simulink model "Test_Counter_4bit_Cfg"  (R2023a)
settings: Solver=VariableStepAuto  StartTime=0.0  StopTime=1000.0  MaxStep=1  MinStep=1  RelTol=1e-3  EnableMultiTasking=on
libraries: simulink x2, simulink_extras x1, Counters_Lib x1
settings Model: PauseTimes=0  Creator=Jozko Mrkvicka  LastModifiedBy=Jozko Mrkvicka
settings SolverCC: InitialStep=1  AlgebraicLoopSolver=TrustRegion
settings DataIOCC: ReturnWorkspaceOutputs=off
settings OptimizationCC: LifeSpan=inf
settings DebuggingCC: UnconnectedInputMsg=warning  UnconnectedOutputMsg=warning  UnconnectedLineMsg=warning  SFUnexpectedBacktrackingDiag=warning  SFNoUnconditionalDefaultTransitionDiag=warning  ArithmeticOperatorsInVariantConditions=warning
settings ModelReferenceCC: EnableRefExpFcnMdlSchedulingChecks=on
settings SFSimCC: SimUseLocalCustomCode=off  CustomCodeUndefinedFunction=UseInterfaceOnly
settings RTWCC: RTWUseLocalCustomCode=off
settings CodeAppCC: StateflowObjectComments=on
settings GRTTargetCC: TargetLangStandard=C89/C90 (ANSI)
settings ConfigComp: CovMetricSettings=dw  CovSaveCumulativeToWorkspaceVar=on  CovSaveSingleToWorkspaceVar=on  CovExternalEMLEnable=off

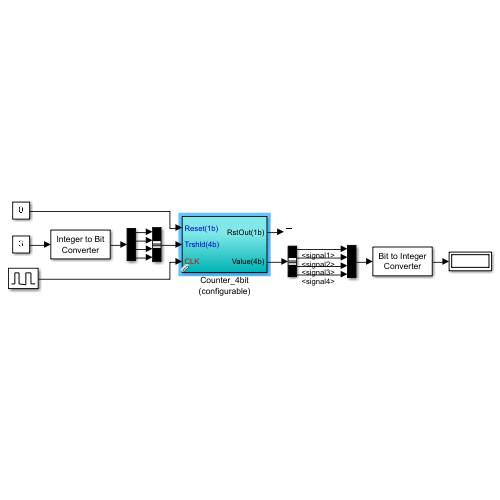
[thumbnail: Simulink's stored preview of the top-level diagram]
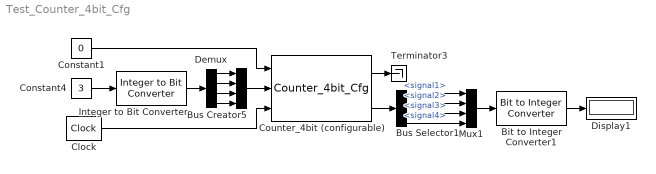
== system Test_Counter_4bit_Cfg ==
  Bit to Integer Converter1 : simulink/Logic and Bit Operations/Bit to Integer Converter  nbits=4  bitOrder=MSB first  signedOutputValues=Unsigned  outDtype=uint8  outDtypeSigned=Inherit via internal rule
      settings: LibrarySourceBlock=|
      | commutil2/Bit to Integer
      | Converter
  Bus Creator5 : BusCreator  Inputs=4
  Bus Selector1 : BusSelector  OutputSignals=signal1,signal2,signal3,signal4
  Clock : simulink_extras/Flip Flops/Clock  period=2
  Constant1 : Constant  Value=0  OutDataTypeStr=boolean
  Constant4 : Constant  Value=3
  Counter_4bit (configurable) : Counters_Lib/Counter_4bit_Cfg  SystemSampleTime=-1  VariantActivationTime=update diagram  Latency=0  AutoFrameSizeCalculation=off
  Demux : Demux
  Display1 : Display
  Integer to Bit Converter : simulink/Logic and Bit Operations/Integer to Bit Converter  nbits=4  signedInputValues=Unsigned  bitOrder=MSB first  outDtype=Inherit via internal rule
      settings: LibrarySourceBlock=|
      | commutil2/Integer to Bit
      | Converter
  Mux1 : Mux
  Terminator3 : Terminator
  wires:
  Mux1/1 -> Bit to Integer Converter1/1
  Bit to Integer Converter1/1 -> Display1/1
  Constant4/1 -> Integer to Bit Converter/1
  Integer to Bit Converter/1 -> Demux/1
  Clock/1 -> Counter_4bit (configurable)/3
  Bus Creator5/1 -> Counter_4bit (configurable)/2
  Constant1/1 -> Counter_4bit (configurable)/1
  Counter_4bit (configurable)/1 -> Terminator3/1
  Counter_4bit (configurable)/2 -> Bus Selector1/1
  Bus Selector1/2 -> Mux1/2  "<signal2>"
  Bus Selector1/3 -> Mux1/3  "<signal3>"
  Bus Selector1/4 -> Mux1/4  "<signal4>"
  Bus Selector1/1 -> Mux1/1  "<signal1>"
  Demux/1 -> Bus Creator5/1
  Demux/2 -> Bus Creator5/2
  Demux/3 -> Bus Creator5/3
  Demux/4 -> Bus Creator5/4
